simulink model "generic_RLC"  (R2014b)
settings: Solver=VariableStepAuto  StartTime=0.0  StopTime=0.2  MaxStep=0.001  RelTol=1e-3
values from neighbouring files (symbols this model uses):
  Mu = [0;0]    [call_generic_01a.m]    (also in call_generic_01b.m; call_generic_02.m = zeros(6,1); call_generic_02N.m = [0;0;0;0;0;0])
  Mw = [0  0  1/C1 ... (first row only)    [call_generic_01a.m]    (also in call_generic_01b.m = [0  0  1/C2; call_generic_02.m = zeros(6,11); call_generic_02N.m = zeros(6,11))
  Mx = zeros(2,2)    [call_generic_01a.m]    (also in call_generic_01b.m; call_generic_02.m = zeros(6,6); call_generic_02N.m = zeros(6,6))
  Nu = [ ... (first row only)    [call_generic_01a.m]    (also in call_generic_01b.m; call_generic_02.m = zeros(11,1); call_generic_02N.m = [1;0;0;0;0;0;0;0;0;0;0])
  Nwi = inv(Nw)    [call_generic_01a.m]    (also in call_generic_01b.m; call_generic_02.m; call_generic_02N.m)
  Nx = [1  0 ... (first row only)    [call_generic_01a.m]    (also in call_generic_01b.m = [0  0; call_generic_02.m = zeros(11,6); call_generic_02N.m = zeros(11,6))
  Pi1 = [0  0;0  0;0  1]    [call_generic_01a.m]    (also in call_generic_01b.m = [0  0;0  1;0  0]; call_generic_02.m = zeros(11,6); call_generic_02N.m = zeros(11,6))
  Pi2 = [0  1  0 ... (first row only)    [call_generic_01a.m]    (also in call_generic_01b.m; call_generic_02.m = zeros(11,11); call_generic_02N.m = zeros(11,11))
  Pv1 = [1  0 ... (first row only)    [call_generic_01a.m]    (also in call_generic_01b.m = [0  0; call_generic_02.m = zeros(6,6); call_generic_02N.m = zeros(6,6))
  Pv2 = [0  0  0 ... (first row only)    [call_generic_01a.m]    (also in call_generic_01b.m = [1  0  0; call_generic_02.m = zeros(6,11); call_generic_02N.m = zeros(6,11))
settings Model: Creator=mchsswh3  LastModifiedBy=Will
settings DataIOCC: LimitDataPoints=off  SaveFormat=Dataset
settings OptimizationCC: UseDivisionForNetSlopeComputation=off  LifeSpan=auto  SimCompilerOptimization=off
settings DebuggingCC: SolverPrmCheckMsg=none  FcnCallInpInsideContextMsg=error  FrameProcessingCompatibilityMsg=error  SFUnexpectedBacktrackingDiag=error  SFNoUnconditionalDefaultTransitionDiag=error
settings HardwareCC: ProdBitPerPointer=64  ProdLargestAtomicFloat=Float  ProdIntDivRoundTo=Zero  ProdEndianess=LittleEndian  ProdWordSize=64  ProdHWDeviceType=Intel->x86-64 (Windows64)
settings ModelReferenceCC: PropagateSignalLabelsOutOfModel=on
settings RTWCC: RTWCompilerOptimization=off
settings GRTTargetCC: TargetLangStandard=C99 (ISO)  GeneratePreprocessorConditionals=Use local settings

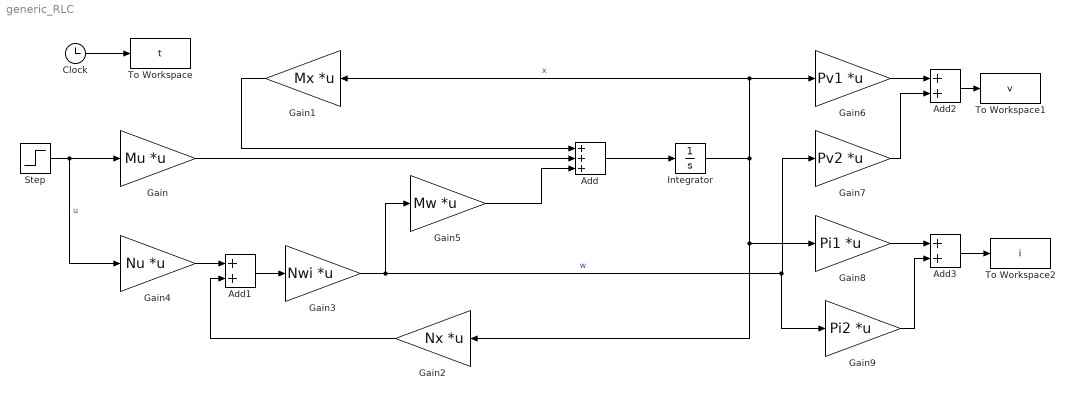
== system generic_RLC ==
  Add : Sum  Inputs=+++
  Add1 : Sum
  Add2 : Sum
  Add3 : Sum
  Clock : Clock
  Gain : Gain  Gain=Mu  Multiplication=Matrix(K*u) (u vector)
  Gain1 : Gain  Gain=Mx  Multiplication=Matrix(K*u) (u vector)
  Gain2 : Gain  Gain=Nx  Multiplication=Matrix(K*u) (u vector)
  Gain3 : Gain  Gain=Nwi  Multiplication=Matrix(K*u) (u vector)
  Gain4 : Gain  Gain=Nu  Multiplication=Matrix(K*u) (u vector)
  Gain5 : Gain  Gain=Mw  Multiplication=Matrix(K*u) (u vector)
  Gain6 : Gain  Gain=Pv1  Multiplication=Matrix(K*u) (u vector)
  Gain7 : Gain  Gain=Pv2  Multiplication=Matrix(K*u) (u vector)
  Gain8 : Gain  Gain=Pi1  Multiplication=Matrix(K*u) (u vector)
  Gain9 : Gain  Gain=Pi2  Multiplication=Matrix(K*u) (u vector)
  Integrator : Integrator
  Step : Step  Time=0  SampleTime=0
  To Workspace : ToWorkspace  VariableName=t  SampleTime=-1
  To Workspace1 : ToWorkspace  VariableName=v  SampleTime=-1
  To Workspace2 : ToWorkspace  VariableName=i  SampleTime=-1
  wires:
  Clock/1 -> To Workspace/1
  Step/1 -> Gain4/1, Gain/1  "u"
  Add/1 -> Integrator/1
  Gain/1 -> Add/2
  Gain1/1 -> Add/1
  Integrator/1 -> Gain6/1, Gain1/1, Gain8/1, Gain2/1  "x"
  Gain4/1 -> Add1/1
  Gain2/1 -> Add1/2
  Add1/1 -> Gain3/1
  Gain3/1 -> Gain5/1, Gain9/1, Gain7/1  "w"
  Gain5/1 -> Add/3
  Gain6/1 -> Add2/1
  Add2/1 -> To Workspace1/1
  Gain7/1 -> Add2/2
  Gain8/1 -> Add3/1
  Gain9/1 -> Add3/2
  Add3/1 -> To Workspace2/1
